simulink model "ex_7_2"  (Simulink 10.1)
settings: Solver=FixedStepAuto  StartTime=0.0  StopTime=20  FixedStep=0.001  RelTol=1e-3
settings Model: Creator=Paulo Padrao  LastModifiedBy=Paulo Padrao
settings DataIOCC: SaveFormat=Dataset
settings OptimizationCC: LifeSpan=auto
settings DebuggingCC: UnderspecifiedInitializationDetection=Simplified  MergeDetectMultiDrivingBlocksExec=error  SFUnexpectedBacktrackingDiag=error  SFNoUnconditionalDefaultTransitionDiag=error  SFExecutionAtInitializationDiag=warning
settings HardwareCC: ProdBitPerPointer=64  ProdBitPerSizeT=64  ProdBitPerPtrDiffT=64  ProdLargestAtomicFloat=Float  ProdIntDivRoundTo=Zero  ProdEndianess=LittleEndian  ProdWordSize=64  ProdHWDeviceType=Intel->x86-64 (Windows64)
settings ModelReferenceCC: PropagateSignalLabelsOutOfModel=on
settings CodeAppCC: StateflowObjectComments=off
settings GRTTargetCC: TargetLangStandard=C99 (ISO)  CombineOutputUpdateFcns=on  GRTInterface=off
settings ConfigComp: CovMetricSettings=dwe  CovHtmlReporting=off  CovSaveCumulativeToWorkspaceVar=off  CovSaveSingleToWorkspaceVar=off  CovExternalEMLEnable=on

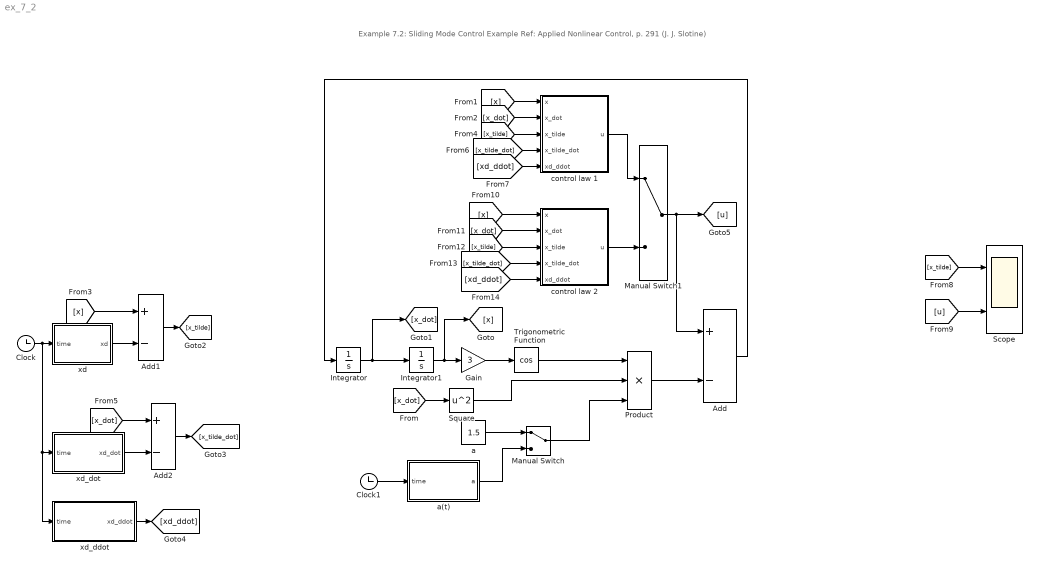
== system ex_7_2 ==
  note: Example 7.2: Sliding Mode Control Example
      | Ref: Applied Nonlinear Control, p. 291 (J. J. Slotine)
  Add : Sum  Inputs=+-
  Add1 : Sum  Inputs=+-
  Add2 : Sum  Inputs=+-
  Clock : Clock
  Clock1 : Clock
  Gain : Gain  Gain=3
  Integrator : Integrator
  Integrator1 : Integrator
  Manual Switch : ManualSwitch
  Manual Switch1 : ManualSwitch
  Product : Product  Inputs=3
  Scope : Scope  NumInputPorts=2
  Square : Math  Operator=square  SignedPower=on  RndMeth=Zero  SaturateOnIntegerOverflow=on
  Trigonometric Function : Trigonometry  Operator=cos
  a : Constant  Value=1.5
  a(t) : MATLAB Function  TreatAsAtomicUnit=on
  control law 1 : Subsystem
  control law 2 : Subsystem
  xd : MATLAB Function  TreatAsAtomicUnit=on
  xd_ddot : MATLAB Function  TreatAsAtomicUnit=on
  xd_dot : MATLAB Function  TreatAsAtomicUnit=on
  wires:
  Integrator/1 -> [x_dot], Integrator1/1
  Gain/1 -> Trigonometric Function/1
  Integrator1/1 -> [x], Gain/1
  Product/1 -> Add/2
  Trigonometric Function/1 -> Product/1
  Square/1 -> Product/2
  Add/1 -> Integrator/1
  Clock/1 -> xd_ddot/1(time), xd_dot/1(time), xd/1(time)
  [x_dot] -> Square/1
  [x] -> control law 1/1(x)
  [x_dot] -> control law 1/2(x_dot)
  xd/1(xd) -> Add1/2
  [x] -> Add1/1
  Add1/1 -> [x_tilde]
  [x_tilde] -> control law 1/3(x_tilde)
  xd_dot/1(xd_dot) -> Add2/2
  Add2/1 -> [x_tilde_dot]
  [x_dot] -> Add2/1
  [x_tilde_dot] -> control law 1/4(x_tilde_dot)
  xd_ddot/1(xd_ddot) -> [xd_ddot]
  [xd_ddot] -> control law 1/5(xd_ddot)
  [x_tilde] -> Scope/1
  [u] -> Scope/2
  Clock1/1 -> a(t)/1(time)
  a/1 -> Manual Switch/1
  Manual Switch/1 -> Product/3
  a(t)/1(a) -> Manual Switch/2
  control law 1/1(u) -> Manual Switch1/1
  [xd_ddot] -> control law 2/5(xd_ddot)
  [x_tilde_dot] -> control law 2/4(x_tilde_dot)
  [x_tilde] -> control law 2/3(x_tilde)
  [x_dot] -> control law 2/2(x_dot)
  [x] -> control law 2/1(x)
  control law 2/1(u) -> Manual Switch1/2
  Manual Switch1/1 -> Add/1, [u]

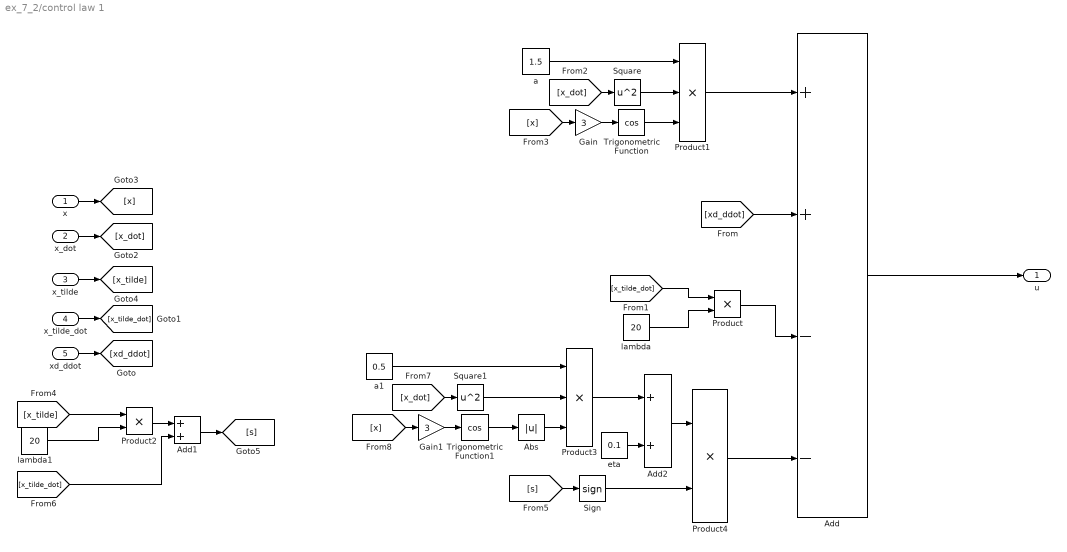
== system ex_7_2/control law 1 ==
  x : Inport
  x_dot : Inport  Port=2
  x_tilde : Inport  Port=3
  x_tilde_dot : Inport  Port=4
  xd_ddot : Inport  Port=5
  Abs : Abs
  Add : Sum  Inputs=++--
  Add1 : Sum
  Add2 : Sum
  Gain : Gain  Gain=3
  Gain1 : Gain  Gain=3
  Product : Product
  Product1 : Product  Inputs=3
  Product2 : Product
  Product3 : Product  Inputs=3
  Product4 : Product
  Sign : Signum  ZeroCross=off
  Square : Math  Operator=square  SignedPower=on  RndMeth=Zero  SaturateOnIntegerOverflow=on
  Square1 : Math  Operator=square  SignedPower=on  RndMeth=Zero  SaturateOnIntegerOverflow=on
  Trigonometric Function : Trigonometry  Operator=cos
  Trigonometric Function1 : Trigonometry  Operator=cos
  a : Constant  Value=1.5
  a1 : Constant  Value=0.5
  eta : Constant  Value=0.1
  lambda : Constant  Value=20
  lambda1 : Constant  Value=20
  u : Outport  VectorParamsAs1DForOutWhenUnconnected=off
  wires:
  Add/1 -> u/1
  xd_ddot/1 -> [xd_ddot]
  [xd_ddot] -> Add/2
  x_tilde_dot/1 -> [x_tilde_dot]
  Product/1 -> Add/3
  [x_tilde_dot] -> Product/1
  lambda/1 -> Product/2
  x_dot/1 -> [x_dot]
  x/1 -> [x]
  x_tilde/1 -> [x_tilde]
  [x_dot] -> Square/1
  Square/1 -> Product1/2
  a/1 -> Product1/1
  [x] -> Gain/1
  Gain/1 -> Trigonometric Function/1
  Trigonometric Function/1 -> Product1/3
  Product1/1 -> Add/1
  [x_tilde] -> Product2/1
  Product2/1 -> Add1/1
  Add1/1 -> [s]
  lambda1/1 -> Product2/2
  [x_tilde_dot] -> Add1/2
  Trigonometric Function1/1 -> Abs/1
  Gain1/1 -> Trigonometric Function1/1
  [x] -> Gain1/1
  a1/1 -> Product3/1
  Square1/1 -> Product3/2
  [x_dot] -> Square1/1
  Product3/1 -> Add2/1
  eta/1 -> Add2/2
  Abs/1 -> Product3/3
  Add2/1 -> Product4/1
  [s] -> Sign/1
  Sign/1 -> Product4/2
  Product4/1 -> Add/4

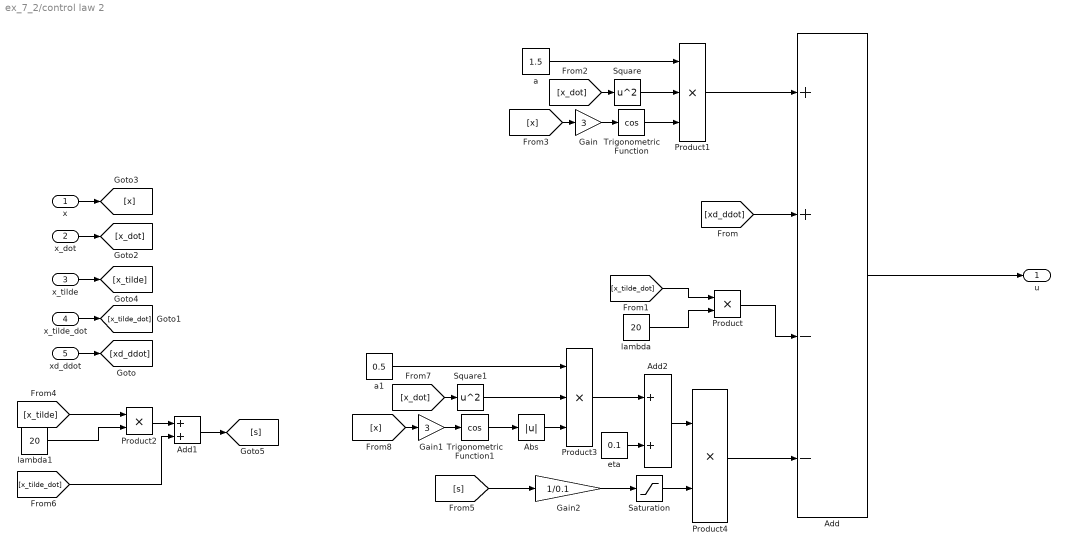
== system ex_7_2/control law 2 ==
  x : Inport
  x_dot : Inport  Port=2
  x_tilde : Inport  Port=3
  x_tilde_dot : Inport  Port=4
  xd_ddot : Inport  Port=5
  Abs : Abs
  Add : Sum  Inputs=++--
  Add1 : Sum
  Add2 : Sum
  Gain : Gain  Gain=3
  Gain1 : Gain  Gain=3
  Gain2 : Gain  Gain=1/0.1
  Product : Product
  Product1 : Product  Inputs=3
  Product2 : Product
  Product3 : Product  Inputs=3
  Product4 : Product
  Saturation : Saturate  UpperLimit=0.1  LowerLimit=-0.1  LinearizeAsGain=off
  Square : Math  Operator=square  SignedPower=on  RndMeth=Zero  SaturateOnIntegerOverflow=on
  Square1 : Math  Operator=square  SignedPower=on  RndMeth=Zero  SaturateOnIntegerOverflow=on
  Trigonometric Function : Trigonometry  Operator=cos
  Trigonometric Function1 : Trigonometry  Operator=cos
  a : Constant  Value=1.5
  a1 : Constant  Value=0.5
  eta : Constant  Value=0.1
  lambda : Constant  Value=20
  lambda1 : Constant  Value=20
  u : Outport  VectorParamsAs1DForOutWhenUnconnected=off
  wires:
  Product4/1 -> Add/4
  Saturation/1 -> Product4/2
  [s] -> Gain2/1
  Add2/1 -> Product4/1
  Abs/1 -> Product3/3
  eta/1 -> Add2/2
  Product3/1 -> Add2/1
  [x_dot] -> Square1/1
  Square1/1 -> Product3/2
  a1/1 -> Product3/1
  [x] -> Gain1/1
  Gain1/1 -> Trigonometric Function1/1
  Trigonometric Function1/1 -> Abs/1
  [x_tilde_dot] -> Add1/2
  lambda1/1 -> Product2/2
  Add1/1 -> [s]
  Product2/1 -> Add1/1
  [x_tilde] -> Product2/1
  Product1/1 -> Add/1
  Trigonometric Function/1 -> Product1/3
  Gain/1 -> Trigonometric Function/1
  [x] -> Gain/1
  a/1 -> Product1/1
  Square/1 -> Product1/2
  [x_dot] -> Square/1
  x_tilde/1 -> [x_tilde]
  x/1 -> [x]
  x_dot/1 -> [x_dot]
  lambda/1 -> Product/2
  [x_tilde_dot] -> Product/1
  Product/1 -> Add/3
  x_tilde_dot/1 -> [x_tilde_dot]
  [xd_ddot] -> Add/2
  xd_ddot/1 -> [xd_ddot]
  Add/1 -> u/1
  Gain2/1 -> Saturation/1

== matlab function xd ==
  data: time input double; xd output double
function xd = fcn(time)

xd = sin(pi*0.5*time);

== matlab function xd_dot ==
  data: time input double; xd_dot output double
function xd_dot = fcn(time)

xd_dot = 0.5*pi*cos((pi/2)*time);

== matlab function xd_ddot ==
  data: time input double; xd_ddot output double
function xd_ddot = fcn(time)

xd_ddot = -0.25*pi^2*sin((pi/2)*time);

== matlab function a(t) ==
  data: time input double; a output double
function a = fcn(time)

a =abs(sin(time)) + 1;
